simulink model "ModeloCC"  (R2021b)
settings: Solver=VariableStepAuto  StartTime=0.0  StopTime=10.0  RelTol=1e-3
undefined symbols (not defined in the file): denMotorsim, numMotorsim
settings Model: Creator=Esther  LastModifiedBy=Esther

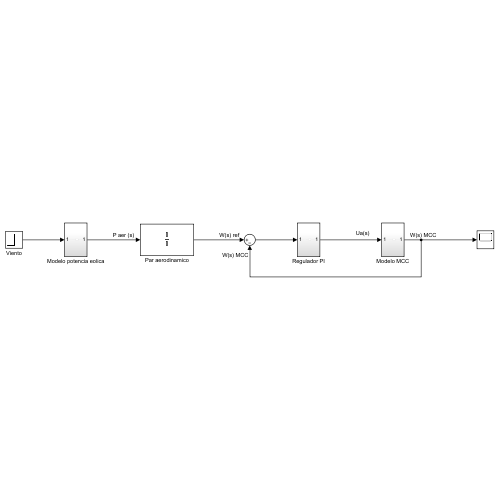
[thumbnail: Simulink's stored preview of the top-level diagram]
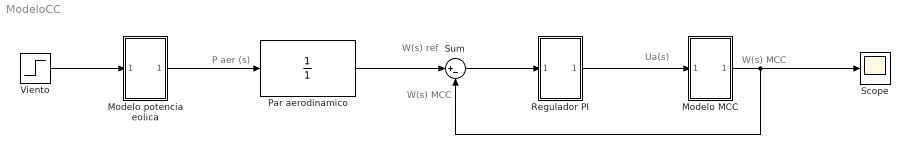
== system ModeloCC ==
  note: Ua(s)
  note: W(s) MCC
  note: W(s) ref
  note: W(s) MCC
  note: P aer (s)
  Modelo MCC : Subsystem
  Modelo potencia eolica : Subsystem
  Par aerodinamico : TransferFcn  Denominator=[1]
  Regulador PI : Subsystem
  Scope : Scope
  Sum : Sum  Inputs=|+-
  Viento : Step  SampleTime=0
  wires:
  Regulador PI/1(Out1) -> Modelo MCC/1(In2)
  Sum/1 -> Regulador PI/1(In2)
  Modelo MCC/1(Out1) -> Sum/2, Scope/1
  Par aerodinamico/1 -> Sum/1
  Modelo potencia eolica/1(Out1) -> Par aerodinamico/1
  Viento/1 -> Modelo potencia eolica/1(In2)

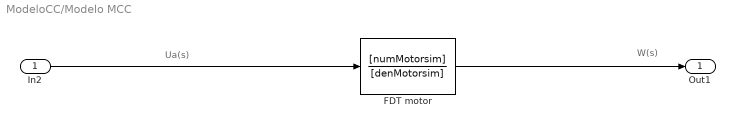
== system ModeloCC/Modelo MCC ==
  note: W(s)
  note: Ua(s)
  In2 : Inport
  FDT motor : TransferFcn  Numerator=[numMotorsim]  Denominator=[denMotorsim]
  Out1 : Outport
  wires:
  FDT motor/1 -> Out1/1
  In2/1 -> FDT motor/1

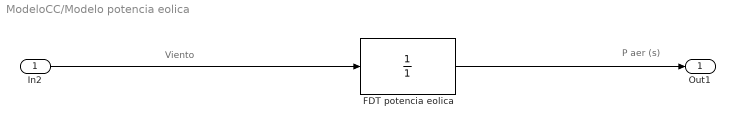
== system ModeloCC/Modelo potencia eolica ==
  note: P aer (s)
  note: Viento
  In2 : Inport
  FDT potencia eolica : TransferFcn  Denominator=[1]
  Out1 : Outport
  wires:
  FDT potencia eolica/1 -> Out1/1
  In2/1 -> FDT potencia eolica/1

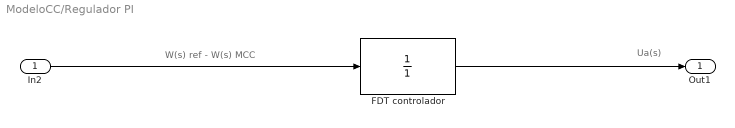
== system ModeloCC/Regulador PI ==
  note: Ua(s)
  note: W(s) ref - W(s) MCC
  In2 : Inport
  FDT controlador : TransferFcn  Denominator=[1]
  Out1 : Outport
  wires:
  FDT controlador/1 -> Out1/1
  In2/1 -> FDT controlador/1
